simulink model "FlightSimulation"  (R2024a)
settings: Solver=VariableStepAuto  StartTime=0.0  StopTime=10.0  RelTol=1e-3
settings Model: Creator=Blind  LastModifiedBy=Blind

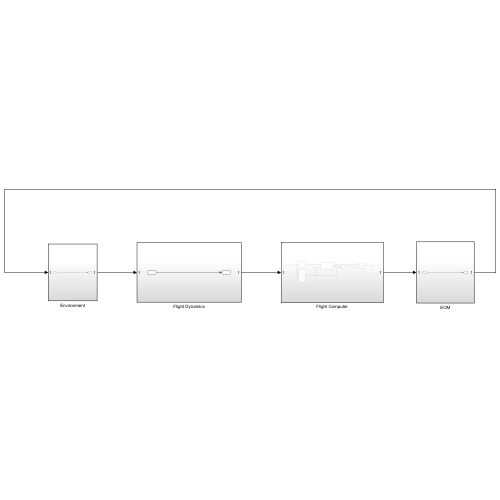
[thumbnail: Simulink's stored preview of the top-level diagram]
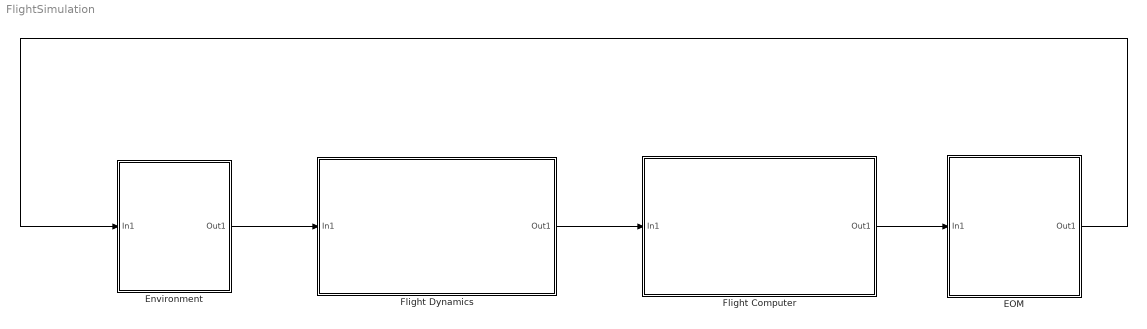
== system FlightSimulation ==
  EOM : Subsystem
  Environment : Subsystem
  Flight Computer : Subsystem
  Flight Dynamics : Subsystem
  wires:
  Flight Dynamics/1(Out1) -> Flight Computer/1(In1)
  Flight Computer/1(Out1) -> EOM/1(In1)
  EOM/1(Out1) -> Environment/1(In1)
  Environment/1(Out1) -> Flight Dynamics/1(In1)

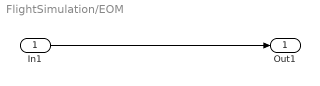
== system FlightSimulation/EOM ==
  In1 : Inport
  Out1 : Outport
  wires:
  In1/1 -> Out1/1

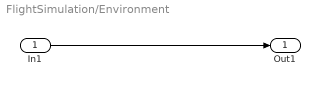
== system FlightSimulation/Environment ==
  In1 : Inport
  Out1 : Outport
  wires:
  In1/1 -> Out1/1

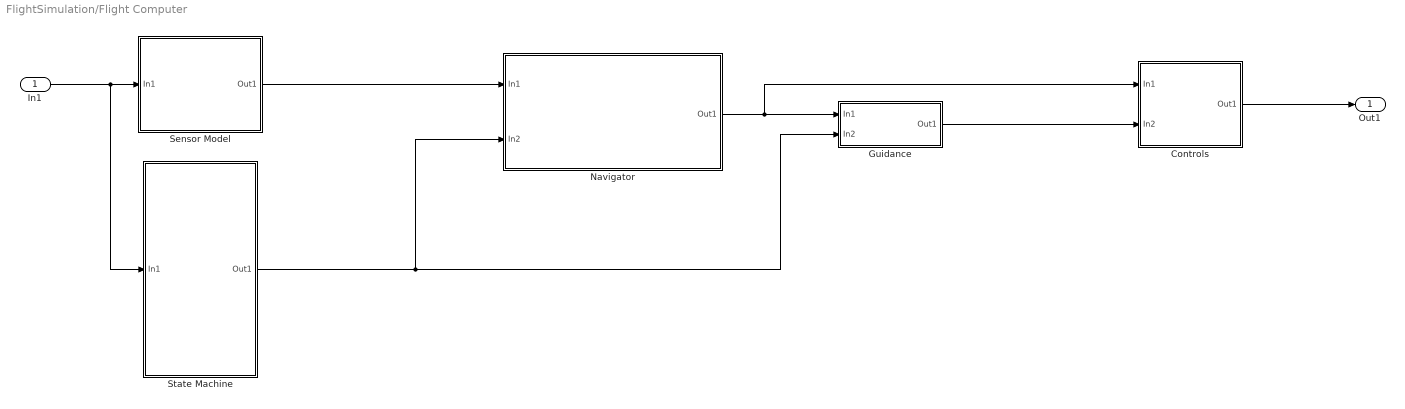
== system FlightSimulation/Flight Computer ==
  In1 : Inport
  Controls : Subsystem
  Guidance : Subsystem
  Navigator : Subsystem
  Sensor Model : Subsystem
  State Machine : Subsystem
  Out1 : Outport
  wires:
  In1/1 -> State Machine/1(In1), Sensor Model/1(In1)
  Sensor Model/1(Out1) -> Navigator/1(In1)
  Guidance/1(Out1) -> Controls/2(In2)
  Navigator/1(Out1) -> Controls/1(In1), Guidance/1(In1)
  State Machine/1(Out1) -> Guidance/2(In2), Navigator/2(In2)
  Controls/1(Out1) -> Out1/1

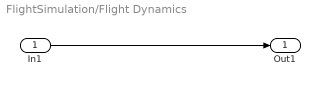
== system FlightSimulation/Flight Dynamics ==
  In1 : Inport
  Out1 : Outport
  wires:
  In1/1 -> Out1/1

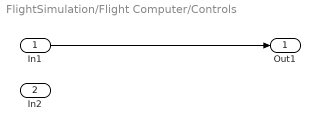
== system FlightSimulation/Flight Computer/Controls ==
  In1 : Inport
  In2 : Inport  Port=2
  Out1 : Outport
  wires:
  In1/1 -> Out1/1

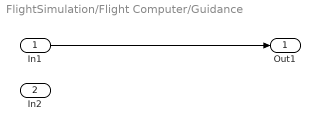
== system FlightSimulation/Flight Computer/Guidance ==
  In1 : Inport
  In2 : Inport  Port=2
  Out1 : Outport
  wires:
  In1/1 -> Out1/1

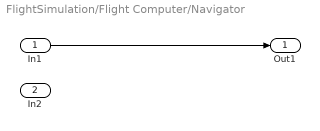
== system FlightSimulation/Flight Computer/Navigator ==
  In1 : Inport
  In2 : Inport  Port=2
  Out1 : Outport
  wires:
  In1/1 -> Out1/1

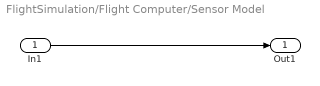
== system FlightSimulation/Flight Computer/Sensor Model ==
  In1 : Inport
  Out1 : Outport
  wires:
  In1/1 -> Out1/1

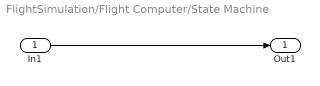
== system FlightSimulation/Flight Computer/State Machine ==
  In1 : Inport
  Out1 : Outport
  wires:
  In1/1 -> Out1/1
